simulink subsystem "sscfluids_ev_battery_cooling_variant"  (R2021b)
settings: Solver=VariableStepAuto  StartTime=0.0  StopTime=10.0  RelTol=1e-3
undefined symbols (not defined in the file): BattTempInit, pipe, pump, radiator, T_env, T_set, tank, valve
libraries: fl_lib x119, nesl_utility x9, SimscapeFluids_lib x7, slpidlib x1, simulink_extras x1
(part 3 of 3)

== system sscfluids_ev_battery_cooling_variant/Cold Plate/One-Pass/Cooling Plate (Pack 2) ==
  Battery to plate conduction : fl_lib/Thermal/Thermal Elements/Conductive Heat Transfer  area=0.5*2 m^2  thickness=1 mm  th_cond=205 W/(m*K)  T_specify=off  T_priority=None  T=0 K  T_nominal_specify=off  T_nominal_unit=K  T_nominal_value=1  Q_specify=off  Q_priority=None  Q=0 W  Q_nominal_specify=off  Q_nominal_unit=W  Q_nominal_value=1
  "Plate mass " : fl_lib/Thermal/Thermal Elements/Thermal Mass  mass=10*2 kg  sp_heat=910 J/kg/K  T_specify=on  T_priority=High  T=BattTempInit degC  T_nominal_specify=off  T_nominal_unit=K  T_nominal_value=1  Q_specify=off  Q_priority=None  Q=0 W  Q_nominal_specify=off  Q_nominal_unit=W  Q_nominal_value=1
  H1 : PMIOPort  Side=Left
  T2 : PMIOPort  Port=2  Side=Right
  connections:
  "Plate mass "/LConn1 -- H1/RConn1 -- Battery to plate conduction/RConn1
  T2/RConn1 -- Battery to plate conduction/LConn1

== system sscfluids_ev_battery_cooling_variant/Cold Plate/One-Pass/Cooling Plate (Pack 3) ==
  Battery to plate conduction : fl_lib/Thermal/Thermal Elements/Conductive Heat Transfer  area=0.5*2 m^2  thickness=1 mm  th_cond=205 W/(m*K)  T_specify=off  T_priority=None  T=0 K  T_nominal_specify=off  T_nominal_unit=K  T_nominal_value=1  Q_specify=off  Q_priority=None  Q=0 W  Q_nominal_specify=off  Q_nominal_unit=W  Q_nominal_value=1
  "Plate mass " : fl_lib/Thermal/Thermal Elements/Thermal Mass  mass=10*2 kg  sp_heat=910 J/kg/K  T_specify=on  T_priority=High  T=BattTempInit degC  T_nominal_specify=off  T_nominal_unit=K  T_nominal_value=1  Q_specify=off  Q_priority=None  Q=0 W  Q_nominal_specify=off  Q_nominal_unit=W  Q_nominal_value=1
  H1 : PMIOPort  Side=Left
  T3 : PMIOPort  Port=2  Side=Right
  connections:
  Battery to plate conduction/LConn1 -- T3/RConn1
  Battery to plate conduction/RConn1 -- H1/RConn1 -- "Plate mass "/LConn1

== system sscfluids_ev_battery_cooling_variant/Cold Plate/One-Pass/Cooling Plate (Pack 4) ==
  Battery to plate conduction : fl_lib/Thermal/Thermal Elements/Conductive Heat Transfer  area=0.5*2 m^2  thickness=1 mm  th_cond=205 W/(m*K)  T_specify=off  T_priority=None  T=0 K  T_nominal_specify=off  T_nominal_unit=K  T_nominal_value=1  Q_specify=off  Q_priority=None  Q=0 W  Q_nominal_specify=off  Q_nominal_unit=W  Q_nominal_value=1
  "Plate mass " : fl_lib/Thermal/Thermal Elements/Thermal Mass  mass=10*2 kg  sp_heat=910 J/kg/K  T_specify=on  T_priority=High  T=BattTempInit degC  T_nominal_specify=off  T_nominal_unit=K  T_nominal_value=1  Q_specify=off  Q_priority=None  Q=0 W  Q_nominal_specify=off  Q_nominal_unit=W  Q_nominal_value=1
  H1 : PMIOPort  Side=Left
  T4 : PMIOPort  Port=2  Side=Right
  connections:
  "Plate mass "/LConn1 -- H1/RConn1 -- Battery to plate conduction/RConn1
  Battery to plate conduction/LConn1 -- T4/RConn1

== system sscfluids_ev_battery_cooling_variant/Cold Plate/Two-Pass/Cooling Plate (Pack 1) ==
  Battery to plate conduction left : fl_lib/Thermal/Thermal Elements/Conductive Heat Transfer  area=0.5 m^2  thickness=1 mm  th_cond=205 W/(m*K)  T_specify=off  T_priority=None  T=0 K  T_nominal_specify=off  T_nominal_unit=K  T_nominal_value=1  Q_specify=off  Q_priority=None  Q=0 W  Q_nominal_specify=off  Q_nominal_unit=W  Q_nominal_value=1
  "Battery to plate conduction right " : fl_lib/Thermal/Thermal Elements/Conductive Heat Transfer  area=0.5 m^2  thickness=1 mm  th_cond=205 W/(m*K)  T_specify=off  T_priority=None  T=0 K  T_nominal_specify=off  T_nominal_unit=K  T_nominal_value=1  Q_specify=off  Q_priority=None  Q=0 W  Q_nominal_specify=off  Q_nominal_unit=W  Q_nominal_value=1
  Cooling channels conduction : fl_lib/Thermal/Thermal Elements/Conductive Heat Transfer  area=1000*0.5 cm^2  thickness=6 cm  th_cond=205 W/(m*K)  T_specify=off  T_priority=None  T=0 K  T_nominal_specify=off  T_nominal_unit=K  T_nominal_value=1  Q_specify=off  Q_priority=None  Q=0 W  Q_nominal_specify=off  Q_nominal_unit=W  Q_nominal_value=1
  "Plate mass left " : fl_lib/Thermal/Thermal Elements/Thermal Mass  mass=10 kg  sp_heat=910 J/kg/K  T_specify=on  T_priority=High  T=BattTempInit degC  T_nominal_specify=off  T_nominal_unit=K  T_nominal_value=1  Q_specify=off  Q_priority=None  Q=0 W  Q_nominal_specify=off  Q_nominal_unit=W  Q_nominal_value=1
  Plate mass right : fl_lib/Thermal/Thermal Elements/Thermal Mass  mass=10 kg  sp_heat=910 J/kg/K  T_specify=on  T_priority=High  T=BattTempInit degC  T_nominal_specify=off  T_nominal_unit=K  T_nominal_value=1  Q_specify=off  Q_priority=None  Q=0 W  Q_nominal_specify=off  Q_nominal_unit=W  Q_nominal_value=1
  H1 : PMIOPort  Side=Left
  H2 : PMIOPort  Port=2  Side=Right
  T1 : PMIOPort  Port=3  Side=Left
  connections:
  Plate mass right/LConn1 -- Cooling channels conduction/RConn1 -- H2/RConn1 -- "Battery to plate conduction right "/RConn1
  T1/RConn1 -- Battery to plate conduction left/LConn1 -- "Battery to plate conduction right "/LConn1
  Battery to plate conduction left/RConn1 -- Cooling channels conduction/LConn1 -- H1/RConn1 -- "Plate mass left "/LConn1

== system sscfluids_ev_battery_cooling_variant/Cold Plate/Two-Pass/Cooling Plate (Pack 2) ==
  Battery to plate conduction left : fl_lib/Thermal/Thermal Elements/Conductive Heat Transfer  area=0.5 m^2  thickness=1 mm  th_cond=205 W/(m*K)  T_specify=off  T_priority=None  T=0 K  T_nominal_specify=off  T_nominal_unit=K  T_nominal_value=1  Q_specify=off  Q_priority=None  Q=0 W  Q_nominal_specify=off  Q_nominal_unit=W  Q_nominal_value=1
  "Battery to plate conduction right " : fl_lib/Thermal/Thermal Elements/Conductive Heat Transfer  area=0.5 m^2  thickness=1 mm  th_cond=205 W/(m*K)  T_specify=off  T_priority=None  T=0 K  T_nominal_specify=off  T_nominal_unit=K  T_nominal_value=1  Q_specify=off  Q_priority=None  Q=0 W  Q_nominal_specify=off  Q_nominal_unit=W  Q_nominal_value=1
  Cooling channels conduction : fl_lib/Thermal/Thermal Elements/Conductive Heat Transfer  area=1000*0.5 cm^2  thickness=6 cm  th_cond=205 W/(m*K)  T_specify=off  T_priority=None  T=0 K  T_nominal_specify=off  T_nominal_unit=K  T_nominal_value=1  Q_specify=off  Q_priority=None  Q=0 W  Q_nominal_specify=off  Q_nominal_unit=W  Q_nominal_value=1
  "Plate mass left " : fl_lib/Thermal/Thermal Elements/Thermal Mass  mass=10 kg  sp_heat=910 J/kg/K  T_specify=on  T_priority=High  T=BattTempInit degC  T_nominal_specify=off  T_nominal_unit=K  T_nominal_value=1  Q_specify=off  Q_priority=None  Q=0 W  Q_nominal_specify=off  Q_nominal_unit=W  Q_nominal_value=1
  Plate mass right : fl_lib/Thermal/Thermal Elements/Thermal Mass  mass=10 kg  sp_heat=910 J/kg/K  T_specify=on  T_priority=High  T=BattTempInit degC  T_nominal_specify=off  T_nominal_unit=K  T_nominal_value=1  Q_specify=off  Q_priority=None  Q=0 W  Q_nominal_specify=off  Q_nominal_unit=W  Q_nominal_value=1
  H1 : PMIOPort  Side=Left
  H2 : PMIOPort  Port=2  Side=Right
  T2 : PMIOPort  Port=3  Side=Left
  connections:
  H1/RConn1 -- "Plate mass left "/LConn1 -- Battery to plate conduction left/RConn1 -- Cooling channels conduction/LConn1
  "Battery to plate conduction right "/LConn1 -- T2/RConn1 -- Battery to plate conduction left/LConn1
  Cooling channels conduction/RConn1 -- "Battery to plate conduction right "/RConn1 -- Plate mass right/LConn1 -- H2/RConn1

== system sscfluids_ev_battery_cooling_variant/Cold Plate/Two-Pass/Cooling Plate (Pack 3) ==
  Battery to plate conduction left : fl_lib/Thermal/Thermal Elements/Conductive Heat Transfer  area=0.5 m^2  thickness=1 mm  th_cond=205 W/(m*K)  T_specify=off  T_priority=None  T=0 K  T_nominal_specify=off  T_nominal_unit=K  T_nominal_value=1  Q_specify=off  Q_priority=None  Q=0 W  Q_nominal_specify=off  Q_nominal_unit=W  Q_nominal_value=1
  "Battery to plate conduction right " : fl_lib/Thermal/Thermal Elements/Conductive Heat Transfer  area=0.5 m^2  thickness=1 mm  th_cond=205 W/(m*K)  T_specify=off  T_priority=None  T=0 K  T_nominal_specify=off  T_nominal_unit=K  T_nominal_value=1  Q_specify=off  Q_priority=None  Q=0 W  Q_nominal_specify=off  Q_nominal_unit=W  Q_nominal_value=1
  Cooling channels conduction : fl_lib/Thermal/Thermal Elements/Conductive Heat Transfer  area=1000*0.5 cm^2  thickness=6 cm  th_cond=205 W/(m*K)  T_specify=off  T_priority=None  T=0 K  T_nominal_specify=off  T_nominal_unit=K  T_nominal_value=1  Q_specify=off  Q_priority=None  Q=0 W  Q_nominal_specify=off  Q_nominal_unit=W  Q_nominal_value=1
  "Plate mass left " : fl_lib/Thermal/Thermal Elements/Thermal Mass  mass=10 kg  sp_heat=910 J/kg/K  T_specify=on  T_priority=High  T=BattTempInit degC  T_nominal_specify=off  T_nominal_unit=K  T_nominal_value=1  Q_specify=off  Q_priority=None  Q=0 W  Q_nominal_specify=off  Q_nominal_unit=W  Q_nominal_value=1
  Plate mass right : fl_lib/Thermal/Thermal Elements/Thermal Mass  mass=10 kg  sp_heat=910 J/kg/K  T_specify=on  T_priority=High  T=BattTempInit degC  T_nominal_specify=off  T_nominal_unit=K  T_nominal_value=1  Q_specify=off  Q_priority=None  Q=0 W  Q_nominal_specify=off  Q_nominal_unit=W  Q_nominal_value=1
  H1 : PMIOPort  Side=Left
  H2 : PMIOPort  Port=2  Side=Right
  T3 : PMIOPort  Port=3  Side=Left
  connections:
  "Plate mass left "/LConn1 -- H1/RConn1 -- Cooling channels conduction/LConn1 -- Battery to plate conduction left/RConn1
  "Battery to plate conduction right "/LConn1 -- Battery to plate conduction left/LConn1 -- T3/RConn1
  "Battery to plate conduction right "/RConn1 -- H2/RConn1 -- Cooling channels conduction/RConn1 -- Plate mass right/LConn1

== system sscfluids_ev_battery_cooling_variant/Cold Plate/Two-Pass/Cooling Plate (Pack 4) ==
  Battery to plate conduction left : fl_lib/Thermal/Thermal Elements/Conductive Heat Transfer  area=0.5 m^2  thickness=1 mm  th_cond=205 W/(m*K)  T_specify=off  T_priority=None  T=0 K  T_nominal_specify=off  T_nominal_unit=K  T_nominal_value=1  Q_specify=off  Q_priority=None  Q=0 W  Q_nominal_specify=off  Q_nominal_unit=W  Q_nominal_value=1
  "Battery to plate conduction right " : fl_lib/Thermal/Thermal Elements/Conductive Heat Transfer  area=0.5 m^2  thickness=1 mm  th_cond=205 W/(m*K)  T_specify=off  T_priority=None  T=0 K  T_nominal_specify=off  T_nominal_unit=K  T_nominal_value=1  Q_specify=off  Q_priority=None  Q=0 W  Q_nominal_specify=off  Q_nominal_unit=W  Q_nominal_value=1
  Cooling channels conduction : fl_lib/Thermal/Thermal Elements/Conductive Heat Transfer  area=1000*0.5 cm^2  thickness=6 cm  th_cond=205 W/(m*K)  T_specify=off  T_priority=None  T=0 K  T_nominal_specify=off  T_nominal_unit=K  T_nominal_value=1  Q_specify=off  Q_priority=None  Q=0 W  Q_nominal_specify=off  Q_nominal_unit=W  Q_nominal_value=1
  "Plate mass left " : fl_lib/Thermal/Thermal Elements/Thermal Mass  mass=10 kg  sp_heat=910 J/kg/K  T_specify=on  T_priority=High  T=BattTempInit degC  T_nominal_specify=off  T_nominal_unit=K  T_nominal_value=1  Q_specify=off  Q_priority=None  Q=0 W  Q_nominal_specify=off  Q_nominal_unit=W  Q_nominal_value=1
  Plate mass right : fl_lib/Thermal/Thermal Elements/Thermal Mass  mass=10 kg  sp_heat=910 J/kg/K  T_specify=on  T_priority=High  T=BattTempInit degC  T_nominal_specify=off  T_nominal_unit=K  T_nominal_value=1  Q_specify=off  Q_priority=None  Q=0 W  Q_nominal_specify=off  Q_nominal_unit=W  Q_nominal_value=1
  H1 : PMIOPort  Side=Left
  H2 : PMIOPort  Port=2  Side=Right
  T4 : PMIOPort  Port=3  Side=Left
  connections:
  Plate mass right/LConn1 -- Cooling channels conduction/RConn1 -- H2/RConn1 -- "Battery to plate conduction right "/RConn1
  T4/RConn1 -- Battery to plate conduction left/LConn1 -- "Battery to plate conduction right "/LConn1
  Battery to plate conduction left/RConn1 -- Cooling channels conduction/LConn1 -- H1/RConn1 -- "Plate mass left "/LConn1

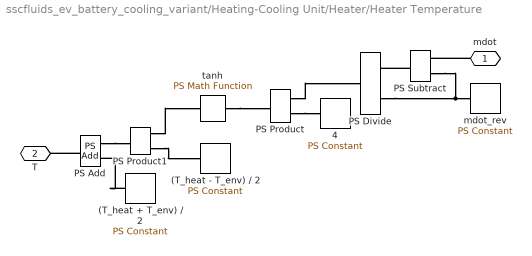
== system sscfluids_ev_battery_cooling_variant/Heating-Cooling Unit/Heater/Heater Temperature ==
  (T_heat + T_env) / 2 : fl_lib/Physical Signals/Sources/PS Constant  constant=(T_heat +T_env + 273.15)/2 K
  (T_heat - T_env) / 2 : fl_lib/Physical Signals/Sources/PS Constant  constant=(T_heat - T_env - 273.15)/2 K
  4 : fl_lib/Physical Signals/Sources/PS Constant  constant=4
  PS Add : fl_lib/Physical Signals/Functions/PS Add
  PS Divide : fl_lib/Physical Signals/Functions/PS Divide
      settings: SourceProductBaseCode=SS
  PS Product : fl_lib/Physical Signals/Functions/PS Product
  PS Product1 : fl_lib/Physical Signals/Functions/PS Product
  PS Subtract : fl_lib/Physical Signals/Functions/PS Subtract
  mdot_rev : fl_lib/Physical Signals/Sources/PS Constant  constant=mdot_rev kg/s
  tanh : fl_lib/Physical Signals/Functions/PS Math Function  fcn_choice=foundation.enum.math_function.tanh  v=1
      settings: SourceProductBaseCode=SS
  mdot : PMIOPort  Side=Left
  T : PMIOPort  Port=2  Side=Right
  connections:
  PS Add/RConn1 -- T/RConn1
  tanh/LConn1 -- PS Product/RConn1
  PS Divide/LConn2 -- PS Subtract/LConn2 -- mdot_rev/RConn1
  PS Product/LConn2 -- 4/RConn1
  PS Add/LConn1 -- PS Product1/RConn1
  PS Subtract/RConn1 -- PS Divide/LConn1
  PS Product1/LConn2 -- (T_heat - T_env) / 2/RConn1
  PS Product1/LConn1 -- tanh/RConn1
  PS Product/LConn1 -- PS Divide/RConn1
  (T_heat + T_env) / 2/RConn1 -- PS Add/LConn2
  mdot/RConn1 -- PS Subtract/LConn1

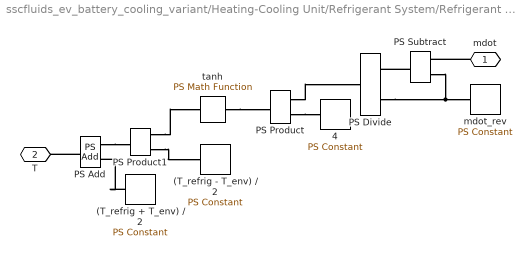
== system sscfluids_ev_battery_cooling_variant/Heating-Cooling Unit/Refrigerant System/Refrigerant Temperature ==
  (T_refrig + T_env) / 2 : fl_lib/Physical Signals/Sources/PS Constant  constant=(T_refrig+T_env+273.15)/2 K
  (T_refrig - T_env) / 2 : fl_lib/Physical Signals/Sources/PS Constant  constant=(T_refrig-T_env-273.15)/2 K
  4 : fl_lib/Physical Signals/Sources/PS Constant  constant=4
  PS Add : fl_lib/Physical Signals/Functions/PS Add
  PS Divide : fl_lib/Physical Signals/Functions/PS Divide
      settings: SourceProductBaseCode=SS
  PS Product : fl_lib/Physical Signals/Functions/PS Product
  PS Product1 : fl_lib/Physical Signals/Functions/PS Product
  PS Subtract : fl_lib/Physical Signals/Functions/PS Subtract
  mdot_rev : fl_lib/Physical Signals/Sources/PS Constant  constant=mdot_rev kg/s
  tanh : fl_lib/Physical Signals/Functions/PS Math Function  fcn_choice=foundation.enum.math_function.tanh  v=1
      settings: SourceProductBaseCode=SS
  mdot : PMIOPort  Side=Left
  T : PMIOPort  Port=2  Side=Right
  connections:
  tanh/LConn1 -- PS Product/RConn1
  PS Product/LConn1 -- PS Divide/RConn1
  (T_refrig + T_env) / 2/RConn1 -- PS Add/LConn2
  PS Divide/LConn2 -- PS Subtract/LConn2 -- mdot_rev/RConn1
  PS Add/RConn1 -- T/RConn1
  PS Add/LConn1 -- PS Product1/RConn1
  PS Product1/LConn1 -- tanh/RConn1
  PS Product/LConn2 -- 4/RConn1
  PS Subtract/RConn1 -- PS Divide/LConn1
  PS Product1/LConn2 -- (T_refrig - T_env) / 2/RConn1
  mdot/RConn1 -- PS Subtract/LConn1
